simulink model "convertGFPower_test"  (R2021a)
settings: Solver=VariableStepAuto  StartTime=0.0  StopTime=10.0  RelTol=1e-3
settings Model: Creator=Jackie Smedley  LastModifiedBy=Jackie Smedley

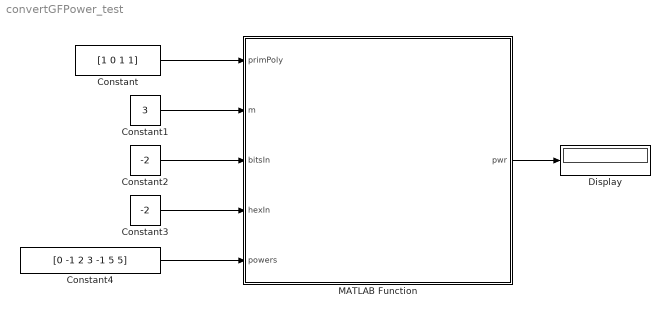
== system convertGFPower_test ==
  Constant : Constant  Value=[1 0 1 1]
  Constant1 : Constant  Value=3
  Constant2 : Constant  Value=-2
  Constant3 : Constant  Value=-2
  Constant4 : Constant  Value=[0 -1 2 3 -1 5 5]
  Display : Display
  MATLAB Function : MATLAB Function  TreatAsAtomicUnit=on
  wires:
  MATLAB Function/1(pwr) -> Display/1
  Constant/1 -> MATLAB Function/1(primPoly)
  Constant1/1 -> MATLAB Function/2(m)
  Constant2/1 -> MATLAB Function/3(bitsIn)
  Constant3/1 -> MATLAB Function/4(hexIn)
  Constant4/1 -> MATLAB Function/5(powers)

== matlab function convertGFPower_test/MATLAB Function ==
  data: primPoly input; pwr output; m input; bitsIn input; hexIn input; powers input
function pwr  = convertGFPowerScript(primPoly, m, bitsIn, hexIn, powers)
gf = GenerateGF2m(primPoly, m);
pwr = convertGFPower(gf, bitsIn, hexIn, powers);
end
